simulink model "ModelSFwithScaling"  (R2019b)
settings: Solver=VariableStepAuto  StartTime=0.0  StopTime=10.0  RelTol=1e-3
values from neighbouring files (symbols this model uses):
  A = [0 -th2 th4; 0 -1/th3 0; 0 0 -1/th5]    [AP_TimeDelay.m]    (also in SmithControl.m; TimeDelayParameters.m = [0 -th2 0 th4 0; 0 -1/th3 1/th3 0 0; 0 0 -1/th3 0 0; 0 0 0 -; positivity_matrix.m; rscale.m = [0 -th2 0 th4 0; 0 -1/th3 1/th3 0 0; 0 0 -1/th3 0 0; 0 0 0 -)
  B = [0 0; 1/th3 0; 0 1/th5]    [AP_TimeDelay.m]    (also in SmithControl.m; TimeDelayParameters.m = [0 0; 0 0; 1/th3 0; 0 0; 0 1/th5]; positivity_matrix.m; rscale.m = [0 0; 0 0; 1/th3 0; 0 0; 0 1/th5])
  Bc = [th1; 0; 0; 0; 0]    [TimeDelayParameters.m]    (also in rscale.m)
  C = [1 1 1]    [AP_TimeDelay.m]    (also in SmithControl.m = [1 0 0]; TimeDelayParameters.m = [1 0 0 0 0]; positivity_matrix.m = [1 0 0]; rscale.m = [1 0 0 0 0])
  Fin = k*[1/th2 -th3 -th3 2 2]    [TimeDelayParameters.m]
  th1 = 0.85    [AP_TimeDelay.m]    (also in SmithControl.m; TimeDelayParameters.m = 0.32; positivity_matrix.m; rscale.m)
  th2 = 50    [AP_TimeDelay.m]    (also in SmithControl.m; TimeDelayParameters.m; positivity_matrix.m; rscale.m)
  x0 = [110; ub; 0]    [AP_TimeDelay.m]    (also in SmithControl.m = [110; ub; ub; 0; 0]; TimeDelayParameters.m = [110; ub; ub; 0; 0]; positivity_matrix.m = [110; th1/th2; 0])
libraries: dspsrcs4 x1
settings Model: Creator=akshita_jain  LastModifiedBy=akshita_jain

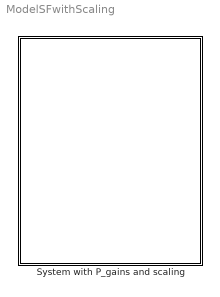
== system ModelSFwithScaling ==
  System with P_gains and scaling : Subsystem

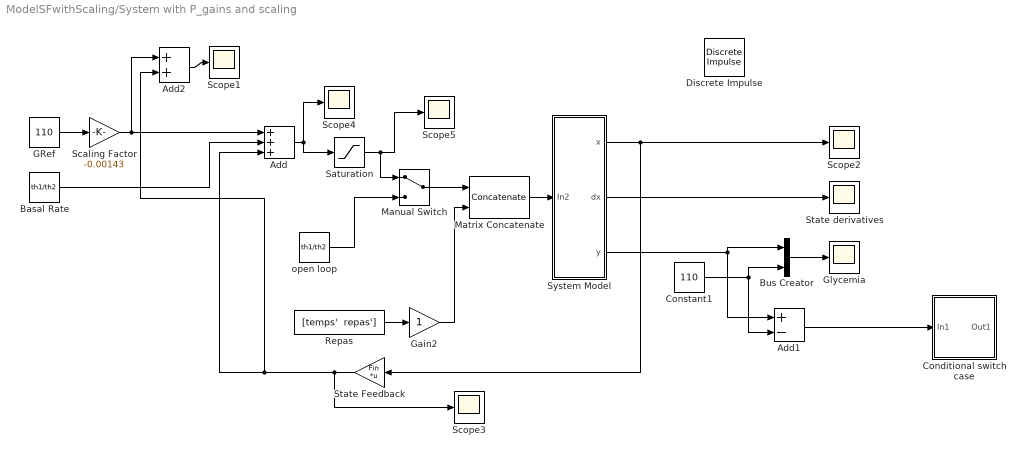
== system ModelSFwithScaling/System with P_gains and scaling ==
  Add : Sum  Inputs=+++
  Add1 : Sum  Inputs=+-
  Add2 : Sum
  Basal Rate : Constant  Value=th1/th2  VectorParams1D=off
  Bus Creator : BusCreator  Inputs=2
  Conditional switch case : Subsystem
  Constant1 : Constant  Value=110
  Discrete Impulse : dspsrcs4/Discrete  Impulse  Delay=100  SampleTime=1  FrameSample=1  OutputFrames=off  dataType=double  isSigned=on  wordLen=16  udDataType=sfix(16)  fracBitsMode=Best precision  numFracBits=15  OutDataTypeStr=double  LastOutDataTypeStr=double
  GRef : Constant  Value=110
  Gain2 : Gain
  Glycemia : Scope
  Manual Switch : ManualSwitch
  Matrix Concatenate : Concatenate  ConcatenateDimension=2
  Repas : FromWorkspace  VariableName="[temps'  repas']"  SampleTime=0
  Saturation : Saturate  UpperLimit=2  LowerLimit=0
  Scaling Factor : Gain  Gain=-0.00143
  Scope{1..5} (5 alike) : Scope
  State Feedback : Gain  Gain=Fin  Multiplication=Matrix(K*u)
  State derivatives : Scope
  System Model : Subsystem
  open loop : Constant  Value=th1/th2
  wires:
  Scaling Factor/1 -> Add2/1, Add/1
  Repas/1 -> Gain2/1
  GRef/1 -> Scaling Factor/1
  Manual Switch/1 -> Matrix Concatenate/1
  Basal Rate/1 -> Add/2
  Add/1 -> Saturation/1, Scope4/1
  Gain2/1 -> Matrix Concatenate/2
  Add2/1 -> Scope1/1
  System Model/1(x) -> State Feedback/1, Scope2/1
  State Feedback/1 -> Add2/2, Add/3, Scope3/1
  System Model/3(y) -> Bus Creator/1, Add1/1
  Add1/1 -> Conditional switch case/1(In1)
  open loop/1 -> Manual Switch/2
  Constant1/1 -> Bus Creator/2, Add1/2
  System Model/2(dx) -> State derivatives/1
  Matrix Concatenate/1 -> System Model/1(In2)
  Saturation/1 -> Manual Switch/1, Scope5/1
  Bus Creator/1 -> Glycemia/1

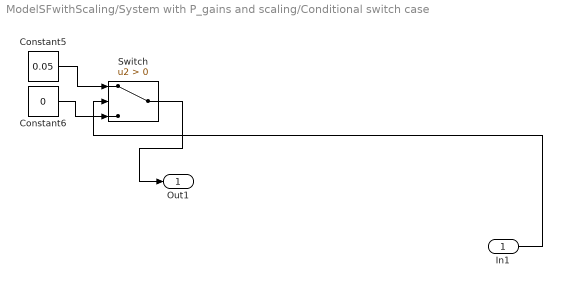
== system ModelSFwithScaling/System with P_gains and scaling/Conditional switch case ==
  In1 : Inport
  Constant5 : Constant  Value=0.05
  Constant6 : Constant  Value=0
  Switch : Switch  Criteria=u2 > Threshold  ZeroCross=off
  Out1 : Outport
  wires:
  In1/1 -> Switch/2
  Constant6/1 -> Switch/3
  Switch/1 -> Out1/1
  Constant5/1 -> Switch/1

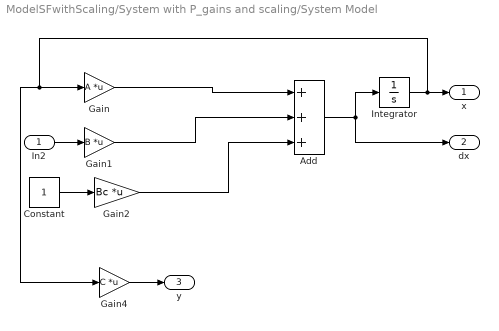
== system ModelSFwithScaling/System with P_gains and scaling/System Model ==
  In2 : Inport
  Add : Sum  Inputs=3
  Constant : Constant
  Gain : Gain  Gain=A  Multiplication=Matrix(K*u)
  Gain1 : Gain  Gain=B  Multiplication=Matrix(K*u)
  Gain2 : Gain  Gain=Bc  Multiplication=Matrix(K*u)
  Gain4 : Gain  Gain=C  Multiplication=Matrix(K*u)
  Integrator : Integrator  InitialCondition=x0  ZeroCross=off
  x : Outport
  dx : Outport  Port=2
  y : Outport  Port=3
  wires:
  Gain2/1 -> Add/3
  Gain/1 -> Add/1
  Constant/1 -> Gain2/1
  Integrator/1 -> Gain4/1, Gain/1, x/1
  In2/1 -> Gain1/1
  Add/1 -> Integrator/1, dx/1
  Gain1/1 -> Add/2
  Gain4/1 -> y/1
